simulink model "Actuator_Models"  (R2025b)
settings: Solver=VariableStepAuto  StartTime=0.0  StopTime=10.0  RelTol=1e-3
undefined symbols (not defined in the file or in its folder): DiscIntNeverNeededParam, distMode, u0
settings Model: DataDictionary=Model_Vars.sldd  Creator=andrew  LastModifiedBy=andrew

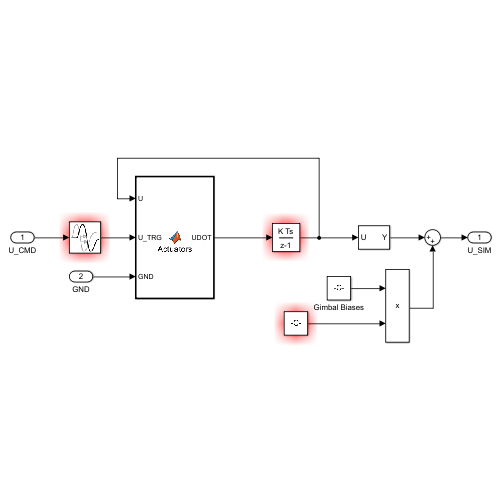
[thumbnail: Simulink's stored preview of the top-level diagram]
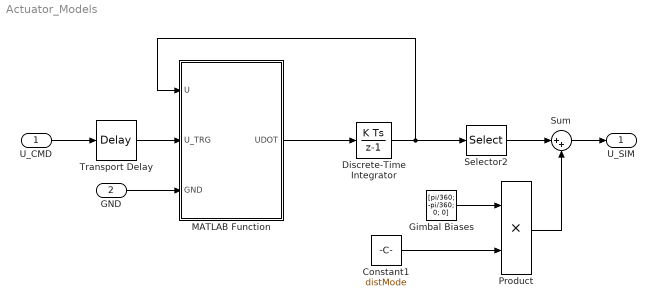
== system Actuator_Models ==
  U_CMD : Inport
  GND : Inport  Port=2
  Constant1 : Constant  Value=distMode
  Discrete-Time Integrator : DiscreteIntegrator  InitialCondition=[zeros(4,1); u0(3); 0]  SampleTime=-1  ICPrevOutput=DiscIntNeverNeededParam  ICPrevScaledInput=DiscIntNeverNeededParam
  Gimbal Biases : Constant  Value=[pi/360; -pi/360; 0; 0]
  MATLAB Function : MATLAB Function  TreatAsAtomicUnit=on
  Product : Product
  Selector2 : Selector  InputPortWidth=6  IndexOptions=Index vector (dialog)  Indices=[1 3 5 6]  OutputSizes=1
  Sum : Sum  Inputs=|++
  Transport Delay : TransportDelay  DelayTime=0.02  InitialOutput=u0
  U_SIM : Outport
  wires:
  Constant1/1 -> Product/2
  Gimbal Biases/1 -> Product/1
  Sum/1 -> U_SIM/1
  MATLAB Function/1(UDOT) -> Discrete-Time Integrator/1
  Selector2/1 -> Sum/1
  Discrete-Time Integrator/1 -> MATLAB Function/1(U), Selector2/1
  GND/1 -> MATLAB Function/3(GND)
  U_CMD/1 -> Transport Delay/1
  Product/1 -> Sum/2
  Transport Delay/1 -> MATLAB Function/2(U_TRG)

== matlab function Actuator_Models/MATLAB Function ==
  data: U input; UDOT output; U_TRG input; GND input
function UDOT = Actuators(U, U_TRG, GND)

    UDOT = ActuatorDynamics(U, U_TRG, GND);
end
